simulink model "c2837xD_lcd_display"  (R2021b)
settings: Solver=FixedStepDiscrete  StartTime=0.0  StopTime=Inf  RelTol=1e-3  EnableMultiTasking=on
InitFcn:
  | c2837xD_Display_Param;
values from neighbouring files (symbols this model uses):
  SCI_counter = SCI_ping_buffer_size/SCI_chunk_size    (= 640)    [c2837xD_Display_Param.m]
  SCI_ping_buffer_size = image_height*lines_in_packet    (= 3840)    [c2837xD_Display_Param.m]
  TI_chunk_size = SCI_chunk_size    (= 6)    [c2837xD_Display_Param.m]
  TI_ping_buffer_size = SCI_ping_buffer_size    (= 3840)    [c2837xD_Display_Param.m]
libraries: c280xlib x63, c2837xDlib x63, simulink x41, c2000lib x1, demo_controls x1, dspswit3 x1, idelinklib_common x1
(part 3 of 4)

== system c2837xD_lcd_display/Initialization/GRAMWindow/Subsystem2/SetData ==
  function : TriggerPort  TriggerType=function-call  VariantControl=Variant
  Constant1 : Constant  SampleTime=-1
  Digital Output1 : c2837xDlib/Digital Output  GPIO_Number=GPIO16~GPIO23  GPIO_Bit0=off  GPIO_BIT0_Toggle=off  GPIO_Bit1=off  GPIO_BIT1_Toggle=off  GPIO_Bit2=off  GPIO_BIT2_Toggle=off  GPIO_Bit3=off  GPIO_BIT3_Toggle=off  GPIO_Bit4=off  GPIO_BIT4_Toggle=off  GPIO_Bit5=off  GPIO_BIT5_Toggle=off  GPIO_Bit6=on  GPIO_BIT6_Toggle=off  GPIO_Bit7=off  GPIO_BIT7_Toggle=off
      settings: SourceProductBaseCode=TIC2000
  wires:
  Constant1/1 -> Digital Output1/1

== system c2837xD_lcd_display/Initialization/GRAMWindow/Subsystem3/SendCommand ==
  cmd : Inport
  function : TriggerPort  TriggerType=function-call  VariantControl=Variant
  SPI Master Transfer : c280xlib/SPI Master Transfer  SPISelect=SPI_A  ClockPolarity=Rising_edge  ClockPhase=Delay_half_cycle  SPIModule=uint32(0)  Mode=Master  BusSpeed=uint32(1000000)  FirstBitToTransfer=Most significant bit (MSB)  ClockMode=0  BlockFunction=Transfer  EnableRegisterAddress=off  RegisterAddress=0  OutputDataType=int8  OutputDataLength=1  DataBits=8  UseCustomSSPin=Explicit GPIO calls  ActiveLowSSPin=Active low  Pin=124
      settings: SourceProductBaseCode=TIC2000
  Terminator : Terminator
  wires:
  cmd/1 -> SPI Master Transfer/1
  SPI Master Transfer/1 -> Terminator/1

== system c2837xD_lcd_display/Initialization/GRAMWindow/Subsystem3/SendData ==
  Data : Inport
  function : TriggerPort  TriggerType=function-call  VariantControl=Variant
  SPI Master Transfer : c280xlib/SPI Master Transfer  SPISelect=SPI_A  ClockPolarity=Rising_edge  ClockPhase=Delay_half_cycle  SPIModule=uint32(0)  Mode=Master  BusSpeed=uint32(1000000)  FirstBitToTransfer=Most significant bit (MSB)  ClockMode=0  BlockFunction=Transfer  EnableRegisterAddress=off  RegisterAddress=0  OutputDataType=int8  OutputDataLength=1  DataBits=8  UseCustomSSPin=Explicit GPIO calls  ActiveLowSSPin=Active low  Pin=124
      settings: SourceProductBaseCode=TIC2000
  Terminator : Terminator
  wires:
  Data/1 -> SPI Master Transfer/1
  SPI Master Transfer/1 -> Terminator/1

== system c2837xD_lcd_display/Initialization/GRAMWindow/Subsystem3/SetCmd ==
  function : TriggerPort  TriggerType=function-call  VariantControl=Variant
  Constant : Constant  Value=0  SampleTime=-1
  Digital Output : c2837xDlib/Digital Output  GPIO_Number=GPIO16~GPIO23  GPIO_Bit0=off  GPIO_BIT0_Toggle=off  GPIO_Bit1=off  GPIO_BIT1_Toggle=off  GPIO_Bit2=off  GPIO_BIT2_Toggle=off  GPIO_Bit3=off  GPIO_BIT3_Toggle=off  GPIO_Bit4=off  GPIO_BIT4_Toggle=off  GPIO_Bit5=off  GPIO_BIT5_Toggle=off  GPIO_Bit6=on  GPIO_BIT6_Toggle=off  GPIO_Bit7=off  GPIO_BIT7_Toggle=off
      settings: SourceProductBaseCode=TIC2000
  wires:
  Constant/1 -> Digital Output/1

== system c2837xD_lcd_display/Initialization/GRAMWindow/Subsystem3/SetData ==
  function : TriggerPort  TriggerType=function-call  VariantControl=Variant
  Constant1 : Constant  SampleTime=-1
  Digital Output1 : c2837xDlib/Digital Output  GPIO_Number=GPIO16~GPIO23  GPIO_Bit0=off  GPIO_BIT0_Toggle=off  GPIO_Bit1=off  GPIO_BIT1_Toggle=off  GPIO_Bit2=off  GPIO_BIT2_Toggle=off  GPIO_Bit3=off  GPIO_BIT3_Toggle=off  GPIO_Bit4=off  GPIO_BIT4_Toggle=off  GPIO_Bit5=off  GPIO_BIT5_Toggle=off  GPIO_Bit6=on  GPIO_BIT6_Toggle=off  GPIO_Bit7=off  GPIO_BIT7_Toggle=off
      settings: SourceProductBaseCode=TIC2000
  wires:
  Constant1/1 -> Digital Output1/1

== system c2837xD_lcd_display/Initialization/GRAMWindow/Subsystem4/SendCommand ==
  cmd : Inport
  function : TriggerPort  TriggerType=function-call  VariantControl=Variant
  SPI Master Transfer : c280xlib/SPI Master Transfer  SPISelect=SPI_A  ClockPolarity=Rising_edge  ClockPhase=Delay_half_cycle  SPIModule=uint32(0)  Mode=Master  BusSpeed=uint32(1000000)  FirstBitToTransfer=Most significant bit (MSB)  ClockMode=0  BlockFunction=Transfer  EnableRegisterAddress=off  RegisterAddress=0  OutputDataType=int8  OutputDataLength=1  DataBits=8  UseCustomSSPin=Explicit GPIO calls  ActiveLowSSPin=Active low  Pin=124
      settings: SourceProductBaseCode=TIC2000
  Terminator : Terminator
  wires:
  cmd/1 -> SPI Master Transfer/1
  SPI Master Transfer/1 -> Terminator/1

== system c2837xD_lcd_display/Initialization/GRAMWindow/Subsystem4/SendData ==
  Data : Inport
  function : TriggerPort  TriggerType=function-call  VariantControl=Variant
  SPI Master Transfer : c280xlib/SPI Master Transfer  SPISelect=SPI_A  ClockPolarity=Rising_edge  ClockPhase=Delay_half_cycle  SPIModule=uint32(0)  Mode=Master  BusSpeed=uint32(1000000)  FirstBitToTransfer=Most significant bit (MSB)  ClockMode=0  BlockFunction=Transfer  EnableRegisterAddress=off  RegisterAddress=0  OutputDataType=int8  OutputDataLength=1  DataBits=8  UseCustomSSPin=Explicit GPIO calls  ActiveLowSSPin=Active low  Pin=124
      settings: SourceProductBaseCode=TIC2000
  Terminator : Terminator
  wires:
  Data/1 -> SPI Master Transfer/1
  SPI Master Transfer/1 -> Terminator/1

== system c2837xD_lcd_display/Initialization/GRAMWindow/Subsystem4/SetCmd ==
  function : TriggerPort  TriggerType=function-call  VariantControl=Variant
  Constant : Constant  Value=0  SampleTime=-1
  Digital Output : c2837xDlib/Digital Output  GPIO_Number=GPIO16~GPIO23  GPIO_Bit0=off  GPIO_BIT0_Toggle=off  GPIO_Bit1=off  GPIO_BIT1_Toggle=off  GPIO_Bit2=off  GPIO_BIT2_Toggle=off  GPIO_Bit3=off  GPIO_BIT3_Toggle=off  GPIO_Bit4=off  GPIO_BIT4_Toggle=off  GPIO_Bit5=off  GPIO_BIT5_Toggle=off  GPIO_Bit6=on  GPIO_BIT6_Toggle=off  GPIO_Bit7=off  GPIO_BIT7_Toggle=off
      settings: SourceProductBaseCode=TIC2000
  wires:
  Constant/1 -> Digital Output/1

== system c2837xD_lcd_display/Initialization/GRAMWindow/Subsystem4/SetData ==
  function : TriggerPort  TriggerType=function-call  VariantControl=Variant
  Constant1 : Constant  SampleTime=-1
  Digital Output1 : c2837xDlib/Digital Output  GPIO_Number=GPIO16~GPIO23  GPIO_Bit0=off  GPIO_BIT0_Toggle=off  GPIO_Bit1=off  GPIO_BIT1_Toggle=off  GPIO_Bit2=off  GPIO_BIT2_Toggle=off  GPIO_Bit3=off  GPIO_BIT3_Toggle=off  GPIO_Bit4=off  GPIO_BIT4_Toggle=off  GPIO_Bit5=off  GPIO_BIT5_Toggle=off  GPIO_Bit6=on  GPIO_BIT6_Toggle=off  GPIO_Bit7=off  GPIO_BIT7_Toggle=off
      settings: SourceProductBaseCode=TIC2000
  wires:
  Constant1/1 -> Digital Output1/1

== system c2837xD_lcd_display/Initialization/GammaCorrection/Subsystem/SendCommand ==
  cmd : Inport
  function : TriggerPort  TriggerType=function-call  VariantControl=Variant
  SPI Master Transfer : c280xlib/SPI Master Transfer  SPISelect=SPI_A  ClockPolarity=Rising_edge  ClockPhase=Delay_half_cycle  SPIModule=uint32(0)  Mode=Master  BusSpeed=uint32(1000000)  FirstBitToTransfer=Most significant bit (MSB)  ClockMode=0  BlockFunction=Transfer  EnableRegisterAddress=off  RegisterAddress=0  OutputDataType=int8  OutputDataLength=1  DataBits=8  UseCustomSSPin=Explicit GPIO calls  ActiveLowSSPin=Active low  Pin=124
      settings: SourceProductBaseCode=TIC2000
  Terminator : Terminator
  wires:
  cmd/1 -> SPI Master Transfer/1
  SPI Master Transfer/1 -> Terminator/1

== system c2837xD_lcd_display/Initialization/GammaCorrection/Subsystem/SendData ==
  Data : Inport
  function : TriggerPort  TriggerType=function-call  VariantControl=Variant
  SPI Master Transfer : c280xlib/SPI Master Transfer  SPISelect=SPI_A  ClockPolarity=Rising_edge  ClockPhase=Delay_half_cycle  SPIModule=uint32(0)  Mode=Master  BusSpeed=uint32(1000000)  FirstBitToTransfer=Most significant bit (MSB)  ClockMode=0  BlockFunction=Transfer  EnableRegisterAddress=off  RegisterAddress=0  OutputDataType=int8  OutputDataLength=1  DataBits=8  UseCustomSSPin=Explicit GPIO calls  ActiveLowSSPin=Active low  Pin=124
      settings: SourceProductBaseCode=TIC2000
  Terminator : Terminator
  wires:
  Data/1 -> SPI Master Transfer/1
  SPI Master Transfer/1 -> Terminator/1

== system c2837xD_lcd_display/Initialization/GammaCorrection/Subsystem/SetCmd ==
  function : TriggerPort  TriggerType=function-call  VariantControl=Variant
  Constant : Constant  Value=0  SampleTime=-1
  Digital Output : c2837xDlib/Digital Output  GPIO_Number=GPIO16~GPIO23  GPIO_Bit0=off  GPIO_BIT0_Toggle=off  GPIO_Bit1=off  GPIO_BIT1_Toggle=off  GPIO_Bit2=off  GPIO_BIT2_Toggle=off  GPIO_Bit3=off  GPIO_BIT3_Toggle=off  GPIO_Bit4=off  GPIO_BIT4_Toggle=off  GPIO_Bit5=off  GPIO_BIT5_Toggle=off  GPIO_Bit6=on  GPIO_BIT6_Toggle=off  GPIO_Bit7=off  GPIO_BIT7_Toggle=off
      settings: SourceProductBaseCode=TIC2000
  wires:
  Constant/1 -> Digital Output/1

== system c2837xD_lcd_display/Initialization/GammaCorrection/Subsystem/SetData ==
  function : TriggerPort  TriggerType=function-call  VariantControl=Variant
  Constant1 : Constant  SampleTime=-1
  Digital Output1 : c2837xDlib/Digital Output  GPIO_Number=GPIO16~GPIO23  GPIO_Bit0=off  GPIO_BIT0_Toggle=off  GPIO_Bit1=off  GPIO_BIT1_Toggle=off  GPIO_Bit2=off  GPIO_BIT2_Toggle=off  GPIO_Bit3=off  GPIO_BIT3_Toggle=off  GPIO_Bit4=off  GPIO_BIT4_Toggle=off  GPIO_Bit5=off  GPIO_BIT5_Toggle=off  GPIO_Bit6=on  GPIO_BIT6_Toggle=off  GPIO_Bit7=off  GPIO_BIT7_Toggle=off
      settings: SourceProductBaseCode=TIC2000
  wires:
  Constant1/1 -> Digital Output1/1

== system c2837xD_lcd_display/Initialization/GammaCorrection/Subsystem1/SendCommand ==
  cmd : Inport
  function : TriggerPort  TriggerType=function-call  VariantControl=Variant
  SPI Master Transfer : c280xlib/SPI Master Transfer  SPISelect=SPI_A  ClockPolarity=Rising_edge  ClockPhase=Delay_half_cycle  SPIModule=uint32(0)  Mode=Master  BusSpeed=uint32(1000000)  FirstBitToTransfer=Most significant bit (MSB)  ClockMode=0  BlockFunction=Transfer  EnableRegisterAddress=off  RegisterAddress=0  OutputDataType=int8  OutputDataLength=1  DataBits=8  UseCustomSSPin=Explicit GPIO calls  ActiveLowSSPin=Active low  Pin=124
      settings: SourceProductBaseCode=TIC2000
  Terminator : Terminator
  wires:
  cmd/1 -> SPI Master Transfer/1
  SPI Master Transfer/1 -> Terminator/1

== system c2837xD_lcd_display/Initialization/GammaCorrection/Subsystem1/SendData ==
  Data : Inport
  function : TriggerPort  TriggerType=function-call  VariantControl=Variant
  SPI Master Transfer : c280xlib/SPI Master Transfer  SPISelect=SPI_A  ClockPolarity=Rising_edge  ClockPhase=Delay_half_cycle  SPIModule=uint32(0)  Mode=Master  BusSpeed=uint32(1000000)  FirstBitToTransfer=Most significant bit (MSB)  ClockMode=0  BlockFunction=Transfer  EnableRegisterAddress=off  RegisterAddress=0  OutputDataType=int8  OutputDataLength=1  DataBits=8  UseCustomSSPin=Explicit GPIO calls  ActiveLowSSPin=Active low  Pin=124
      settings: SourceProductBaseCode=TIC2000
  Terminator : Terminator
  wires:
  Data/1 -> SPI Master Transfer/1
  SPI Master Transfer/1 -> Terminator/1

== system c2837xD_lcd_display/Initialization/GammaCorrection/Subsystem1/SetCmd ==
  function : TriggerPort  TriggerType=function-call  VariantControl=Variant
  Constant : Constant  Value=0  SampleTime=-1
  Digital Output : c2837xDlib/Digital Output  GPIO_Number=GPIO16~GPIO23  GPIO_Bit0=off  GPIO_BIT0_Toggle=off  GPIO_Bit1=off  GPIO_BIT1_Toggle=off  GPIO_Bit2=off  GPIO_BIT2_Toggle=off  GPIO_Bit3=off  GPIO_BIT3_Toggle=off  GPIO_Bit4=off  GPIO_BIT4_Toggle=off  GPIO_Bit5=off  GPIO_BIT5_Toggle=off  GPIO_Bit6=on  GPIO_BIT6_Toggle=off  GPIO_Bit7=off  GPIO_BIT7_Toggle=off
      settings: SourceProductBaseCode=TIC2000
  wires:
  Constant/1 -> Digital Output/1

== system c2837xD_lcd_display/Initialization/GammaCorrection/Subsystem1/SetData ==
  function : TriggerPort  TriggerType=function-call  VariantControl=Variant
  Constant1 : Constant  SampleTime=-1
  Digital Output1 : c2837xDlib/Digital Output  GPIO_Number=GPIO16~GPIO23  GPIO_Bit0=off  GPIO_BIT0_Toggle=off  GPIO_Bit1=off  GPIO_BIT1_Toggle=off  GPIO_Bit2=off  GPIO_BIT2_Toggle=off  GPIO_Bit3=off  GPIO_BIT3_Toggle=off  GPIO_Bit4=off  GPIO_BIT4_Toggle=off  GPIO_Bit5=off  GPIO_BIT5_Toggle=off  GPIO_Bit6=on  GPIO_BIT6_Toggle=off  GPIO_Bit7=off  GPIO_BIT7_Toggle=off
      settings: SourceProductBaseCode=TIC2000
  wires:
  Constant1/1 -> Digital Output1/1

== system c2837xD_lcd_display/Initialization/GammaCorrection/Subsystem2/SendCommand ==
  cmd : Inport
  function : TriggerPort  TriggerType=function-call  VariantControl=Variant
  SPI Master Transfer : c280xlib/SPI Master Transfer  SPISelect=SPI_A  ClockPolarity=Rising_edge  ClockPhase=Delay_half_cycle  SPIModule=uint32(0)  Mode=Master  BusSpeed=uint32(1000000)  FirstBitToTransfer=Most significant bit (MSB)  ClockMode=0  BlockFunction=Transfer  EnableRegisterAddress=off  RegisterAddress=0  OutputDataType=int8  OutputDataLength=1  DataBits=8  UseCustomSSPin=Explicit GPIO calls  ActiveLowSSPin=Active low  Pin=124
      settings: SourceProductBaseCode=TIC2000
  Terminator : Terminator
  wires:
  cmd/1 -> SPI Master Transfer/1
  SPI Master Transfer/1 -> Terminator/1

== system c2837xD_lcd_display/Initialization/GammaCorrection/Subsystem2/SendData ==
  Data : Inport
  function : TriggerPort  TriggerType=function-call  VariantControl=Variant
  SPI Master Transfer : c280xlib/SPI Master Transfer  SPISelect=SPI_A  ClockPolarity=Rising_edge  ClockPhase=Delay_half_cycle  SPIModule=uint32(0)  Mode=Master  BusSpeed=uint32(1000000)  FirstBitToTransfer=Most significant bit (MSB)  ClockMode=0  BlockFunction=Transfer  EnableRegisterAddress=off  RegisterAddress=0  OutputDataType=int8  OutputDataLength=1  DataBits=8  UseCustomSSPin=Explicit GPIO calls  ActiveLowSSPin=Active low  Pin=124
      settings: SourceProductBaseCode=TIC2000
  Terminator : Terminator
  wires:
  Data/1 -> SPI Master Transfer/1
  SPI Master Transfer/1 -> Terminator/1

== system c2837xD_lcd_display/Initialization/GammaCorrection/Subsystem2/SetCmd ==
  function : TriggerPort  TriggerType=function-call  VariantControl=Variant
  Constant : Constant  Value=0  SampleTime=-1
  Digital Output : c2837xDlib/Digital Output  GPIO_Number=GPIO16~GPIO23  GPIO_Bit0=off  GPIO_BIT0_Toggle=off  GPIO_Bit1=off  GPIO_BIT1_Toggle=off  GPIO_Bit2=off  GPIO_BIT2_Toggle=off  GPIO_Bit3=off  GPIO_BIT3_Toggle=off  GPIO_Bit4=off  GPIO_BIT4_Toggle=off  GPIO_Bit5=off  GPIO_BIT5_Toggle=off  GPIO_Bit6=on  GPIO_BIT6_Toggle=off  GPIO_Bit7=off  GPIO_BIT7_Toggle=off
      settings: SourceProductBaseCode=TIC2000
  wires:
  Constant/1 -> Digital Output/1

== system c2837xD_lcd_display/Initialization/GammaCorrection/Subsystem2/SetData ==
  function : TriggerPort  TriggerType=function-call  VariantControl=Variant
  Constant1 : Constant  SampleTime=-1
  Digital Output1 : c2837xDlib/Digital Output  GPIO_Number=GPIO16~GPIO23  GPIO_Bit0=off  GPIO_BIT0_Toggle=off  GPIO_Bit1=off  GPIO_BIT1_Toggle=off  GPIO_Bit2=off  GPIO_BIT2_Toggle=off  GPIO_Bit3=off  GPIO_BIT3_Toggle=off  GPIO_Bit4=off  GPIO_BIT4_Toggle=off  GPIO_Bit5=off  GPIO_BIT5_Toggle=off  GPIO_Bit6=on  GPIO_BIT6_Toggle=off  GPIO_Bit7=off  GPIO_BIT7_Toggle=off
      settings: SourceProductBaseCode=TIC2000
  wires:
  Constant1/1 -> Digital Output1/1

== system c2837xD_lcd_display/Initialization/GammaCorrection/Subsystem3/SendCommand ==
  cmd : Inport
  function : TriggerPort  TriggerType=function-call  VariantControl=Variant
  SPI Master Transfer : c280xlib/SPI Master Transfer  SPISelect=SPI_A  ClockPolarity=Rising_edge  ClockPhase=Delay_half_cycle  SPIModule=uint32(0)  Mode=Master  BusSpeed=uint32(1000000)  FirstBitToTransfer=Most significant bit (MSB)  ClockMode=0  BlockFunction=Transfer  EnableRegisterAddress=off  RegisterAddress=0  OutputDataType=int8  OutputDataLength=1  DataBits=8  UseCustomSSPin=Explicit GPIO calls  ActiveLowSSPin=Active low  Pin=124
      settings: SourceProductBaseCode=TIC2000
  Terminator : Terminator
  wires:
  cmd/1 -> SPI Master Transfer/1
  SPI Master Transfer/1 -> Terminator/1

== system c2837xD_lcd_display/Initialization/GammaCorrection/Subsystem3/SendData ==
  Data : Inport
  function : TriggerPort  TriggerType=function-call  VariantControl=Variant
  SPI Master Transfer : c280xlib/SPI Master Transfer  SPISelect=SPI_A  ClockPolarity=Rising_edge  ClockPhase=Delay_half_cycle  SPIModule=uint32(0)  Mode=Master  BusSpeed=uint32(1000000)  FirstBitToTransfer=Most significant bit (MSB)  ClockMode=0  BlockFunction=Transfer  EnableRegisterAddress=off  RegisterAddress=0  OutputDataType=int8  OutputDataLength=1  DataBits=8  UseCustomSSPin=Explicit GPIO calls  ActiveLowSSPin=Active low  Pin=124
      settings: SourceProductBaseCode=TIC2000
  Terminator : Terminator
  wires:
  Data/1 -> SPI Master Transfer/1
  SPI Master Transfer/1 -> Terminator/1

== system c2837xD_lcd_display/Initialization/GammaCorrection/Subsystem3/SetCmd ==
  function : TriggerPort  TriggerType=function-call  VariantControl=Variant
  Constant : Constant  Value=0  SampleTime=-1
  Digital Output : c2837xDlib/Digital Output  GPIO_Number=GPIO16~GPIO23  GPIO_Bit0=off  GPIO_BIT0_Toggle=off  GPIO_Bit1=off  GPIO_BIT1_Toggle=off  GPIO_Bit2=off  GPIO_BIT2_Toggle=off  GPIO_Bit3=off  GPIO_BIT3_Toggle=off  GPIO_Bit4=off  GPIO_BIT4_Toggle=off  GPIO_Bit5=off  GPIO_BIT5_Toggle=off  GPIO_Bit6=on  GPIO_BIT6_Toggle=off  GPIO_Bit7=off  GPIO_BIT7_Toggle=off
      settings: SourceProductBaseCode=TIC2000
  wires:
  Constant/1 -> Digital Output/1

== system c2837xD_lcd_display/Initialization/GammaCorrection/Subsystem3/SetData ==
  function : TriggerPort  TriggerType=function-call  VariantControl=Variant
  Constant1 : Constant  SampleTime=-1
  Digital Output1 : c2837xDlib/Digital Output  GPIO_Number=GPIO16~GPIO23  GPIO_Bit0=off  GPIO_BIT0_Toggle=off  GPIO_Bit1=off  GPIO_BIT1_Toggle=off  GPIO_Bit2=off  GPIO_BIT2_Toggle=off  GPIO_Bit3=off  GPIO_BIT3_Toggle=off  GPIO_Bit4=off  GPIO_BIT4_Toggle=off  GPIO_Bit5=off  GPIO_BIT5_Toggle=off  GPIO_Bit6=on  GPIO_BIT6_Toggle=off  GPIO_Bit7=off  GPIO_BIT7_Toggle=off
      settings: SourceProductBaseCode=TIC2000
  wires:
  Constant1/1 -> Digital Output1/1

== system c2837xD_lcd_display/Initialization/GammaCorrection/Subsystem4/SendCommand ==
  cmd : Inport
  function : TriggerPort  TriggerType=function-call  VariantControl=Variant
  SPI Master Transfer : c280xlib/SPI Master Transfer  SPISelect=SPI_A  ClockPolarity=Rising_edge  ClockPhase=Delay_half_cycle  SPIModule=uint32(0)  Mode=Master  BusSpeed=uint32(1000000)  FirstBitToTransfer=Most significant bit (MSB)  ClockMode=0  BlockFunction=Transfer  EnableRegisterAddress=off  RegisterAddress=0  OutputDataType=int8  OutputDataLength=1  DataBits=8  UseCustomSSPin=Explicit GPIO calls  ActiveLowSSPin=Active low  Pin=124
      settings: SourceProductBaseCode=TIC2000
  Terminator : Terminator
  wires:
  cmd/1 -> SPI Master Transfer/1
  SPI Master Transfer/1 -> Terminator/1

== system c2837xD_lcd_display/Initialization/GammaCorrection/Subsystem4/SendData ==
  Data : Inport
  function : TriggerPort  TriggerType=function-call  VariantControl=Variant
  SPI Master Transfer : c280xlib/SPI Master Transfer  SPISelect=SPI_A  ClockPolarity=Rising_edge  ClockPhase=Delay_half_cycle  SPIModule=uint32(0)  Mode=Master  BusSpeed=uint32(1000000)  FirstBitToTransfer=Most significant bit (MSB)  ClockMode=0  BlockFunction=Transfer  EnableRegisterAddress=off  RegisterAddress=0  OutputDataType=int8  OutputDataLength=1  DataBits=8  UseCustomSSPin=Explicit GPIO calls  ActiveLowSSPin=Active low  Pin=124
      settings: SourceProductBaseCode=TIC2000
  Terminator : Terminator
  wires:
  Data/1 -> SPI Master Transfer/1
  SPI Master Transfer/1 -> Terminator/1

== system c2837xD_lcd_display/Initialization/GammaCorrection/Subsystem4/SetCmd ==
  function : TriggerPort  TriggerType=function-call  VariantControl=Variant
  Constant : Constant  Value=0  SampleTime=-1
  Digital Output : c2837xDlib/Digital Output  GPIO_Number=GPIO16~GPIO23  GPIO_Bit0=off  GPIO_BIT0_Toggle=off  GPIO_Bit1=off  GPIO_BIT1_Toggle=off  GPIO_Bit2=off  GPIO_BIT2_Toggle=off  GPIO_Bit3=off  GPIO_BIT3_Toggle=off  GPIO_Bit4=off  GPIO_BIT4_Toggle=off  GPIO_Bit5=off  GPIO_BIT5_Toggle=off  GPIO_Bit6=on  GPIO_BIT6_Toggle=off  GPIO_Bit7=off  GPIO_BIT7_Toggle=off
      settings: SourceProductBaseCode=TIC2000
  wires:
  Constant/1 -> Digital Output/1

== system c2837xD_lcd_display/Initialization/GammaCorrection/Subsystem4/SetData ==
  function : TriggerPort  TriggerType=function-call  VariantControl=Variant
  Constant1 : Constant  SampleTime=-1
  Digital Output1 : c2837xDlib/Digital Output  GPIO_Number=GPIO16~GPIO23  GPIO_Bit0=off  GPIO_BIT0_Toggle=off  GPIO_Bit1=off  GPIO_BIT1_Toggle=off  GPIO_Bit2=off  GPIO_BIT2_Toggle=off  GPIO_Bit3=off  GPIO_BIT3_Toggle=off  GPIO_Bit4=off  GPIO_BIT4_Toggle=off  GPIO_Bit5=off  GPIO_BIT5_Toggle=off  GPIO_Bit6=on  GPIO_BIT6_Toggle=off  GPIO_Bit7=off  GPIO_BIT7_Toggle=off
      settings: SourceProductBaseCode=TIC2000
  wires:
  Constant1/1 -> Digital Output1/1

== system c2837xD_lcd_display/Initialization/GammaCorrection1/Subsystem/SendCommand ==
  cmd : Inport
  function : TriggerPort  TriggerType=function-call  VariantControl=Variant
  SPI Master Transfer : c280xlib/SPI Master Transfer  SPISelect=SPI_A  ClockPolarity=Rising_edge  ClockPhase=Delay_half_cycle  SPIModule=uint32(0)  Mode=Master  BusSpeed=uint32(1000000)  FirstBitToTransfer=Most significant bit (MSB)  ClockMode=0  BlockFunction=Transfer  EnableRegisterAddress=off  RegisterAddress=0  OutputDataType=int8  OutputDataLength=1  DataBits=8  UseCustomSSPin=Explicit GPIO calls  ActiveLowSSPin=Active low  Pin=124
      settings: SourceProductBaseCode=TIC2000
  Terminator : Terminator
  wires:
  cmd/1 -> SPI Master Transfer/1
  SPI Master Transfer/1 -> Terminator/1

== system c2837xD_lcd_display/Initialization/GammaCorrection1/Subsystem/SendData ==
  Data : Inport
  function : TriggerPort  TriggerType=function-call  VariantControl=Variant
  SPI Master Transfer : c280xlib/SPI Master Transfer  SPISelect=SPI_A  ClockPolarity=Rising_edge  ClockPhase=Delay_half_cycle  SPIModule=uint32(0)  Mode=Master  BusSpeed=uint32(1000000)  FirstBitToTransfer=Most significant bit (MSB)  ClockMode=0  BlockFunction=Transfer  EnableRegisterAddress=off  RegisterAddress=0  OutputDataType=int8  OutputDataLength=1  DataBits=8  UseCustomSSPin=Explicit GPIO calls  ActiveLowSSPin=Active low  Pin=124
      settings: SourceProductBaseCode=TIC2000
  Terminator : Terminator
  wires:
  Data/1 -> SPI Master Transfer/1
  SPI Master Transfer/1 -> Terminator/1

== system c2837xD_lcd_display/Initialization/GammaCorrection1/Subsystem/SetCmd ==
  function : TriggerPort  TriggerType=function-call  VariantControl=Variant
  Constant : Constant  Value=0  SampleTime=-1
  Digital Output : c2837xDlib/Digital Output  GPIO_Number=GPIO16~GPIO23  GPIO_Bit0=off  GPIO_BIT0_Toggle=off  GPIO_Bit1=off  GPIO_BIT1_Toggle=off  GPIO_Bit2=off  GPIO_BIT2_Toggle=off  GPIO_Bit3=off  GPIO_BIT3_Toggle=off  GPIO_Bit4=off  GPIO_BIT4_Toggle=off  GPIO_Bit5=off  GPIO_BIT5_Toggle=off  GPIO_Bit6=on  GPIO_BIT6_Toggle=off  GPIO_Bit7=off  GPIO_BIT7_Toggle=off
      settings: SourceProductBaseCode=TIC2000
  wires:
  Constant/1 -> Digital Output/1

== system c2837xD_lcd_display/Initialization/GammaCorrection1/Subsystem/SetData ==
  function : TriggerPort  TriggerType=function-call  VariantControl=Variant
  Constant1 : Constant  SampleTime=-1
  Digital Output1 : c2837xDlib/Digital Output  GPIO_Number=GPIO16~GPIO23  GPIO_Bit0=off  GPIO_BIT0_Toggle=off  GPIO_Bit1=off  GPIO_BIT1_Toggle=off  GPIO_Bit2=off  GPIO_BIT2_Toggle=off  GPIO_Bit3=off  GPIO_BIT3_Toggle=off  GPIO_Bit4=off  GPIO_BIT4_Toggle=off  GPIO_Bit5=off  GPIO_BIT5_Toggle=off  GPIO_Bit6=on  GPIO_BIT6_Toggle=off  GPIO_Bit7=off  GPIO_BIT7_Toggle=off
      settings: SourceProductBaseCode=TIC2000
  wires:
  Constant1/1 -> Digital Output1/1

== system c2837xD_lcd_display/Initialization/GammaCorrection1/Subsystem1/SendCommand ==
  cmd : Inport
  function : TriggerPort  TriggerType=function-call  VariantControl=Variant
  SPI Master Transfer : c280xlib/SPI Master Transfer  SPISelect=SPI_A  ClockPolarity=Rising_edge  ClockPhase=Delay_half_cycle  SPIModule=uint32(0)  Mode=Master  BusSpeed=uint32(1000000)  FirstBitToTransfer=Most significant bit (MSB)  ClockMode=0  BlockFunction=Transfer  EnableRegisterAddress=off  RegisterAddress=0  OutputDataType=int8  OutputDataLength=1  DataBits=8  UseCustomSSPin=Explicit GPIO calls  ActiveLowSSPin=Active low  Pin=124
      settings: SourceProductBaseCode=TIC2000
  Terminator : Terminator
  wires:
  cmd/1 -> SPI Master Transfer/1
  SPI Master Transfer/1 -> Terminator/1

== system c2837xD_lcd_display/Initialization/GammaCorrection1/Subsystem1/SendData ==
  Data : Inport
  function : TriggerPort  TriggerType=function-call  VariantControl=Variant
  SPI Master Transfer : c280xlib/SPI Master Transfer  SPISelect=SPI_A  ClockPolarity=Rising_edge  ClockPhase=Delay_half_cycle  SPIModule=uint32(0)  Mode=Master  BusSpeed=uint32(1000000)  FirstBitToTransfer=Most significant bit (MSB)  ClockMode=0  BlockFunction=Transfer  EnableRegisterAddress=off  RegisterAddress=0  OutputDataType=int8  OutputDataLength=1  DataBits=8  UseCustomSSPin=Explicit GPIO calls  ActiveLowSSPin=Active low  Pin=124
      settings: SourceProductBaseCode=TIC2000
  Terminator : Terminator
  wires:
  Data/1 -> SPI Master Transfer/1
  SPI Master Transfer/1 -> Terminator/1

== system c2837xD_lcd_display/Initialization/GammaCorrection1/Subsystem1/SetCmd ==
  function : TriggerPort  TriggerType=function-call  VariantControl=Variant
  Constant : Constant  Value=0  SampleTime=-1
  Digital Output : c2837xDlib/Digital Output  GPIO_Number=GPIO16~GPIO23  GPIO_Bit0=off  GPIO_BIT0_Toggle=off  GPIO_Bit1=off  GPIO_BIT1_Toggle=off  GPIO_Bit2=off  GPIO_BIT2_Toggle=off  GPIO_Bit3=off  GPIO_BIT3_Toggle=off  GPIO_Bit4=off  GPIO_BIT4_Toggle=off  GPIO_Bit5=off  GPIO_BIT5_Toggle=off  GPIO_Bit6=on  GPIO_BIT6_Toggle=off  GPIO_Bit7=off  GPIO_BIT7_Toggle=off
      settings: SourceProductBaseCode=TIC2000
  wires:
  Constant/1 -> Digital Output/1

== system c2837xD_lcd_display/Initialization/GammaCorrection1/Subsystem1/SetData ==
  function : TriggerPort  TriggerType=function-call  VariantControl=Variant
  Constant1 : Constant  SampleTime=-1
  Digital Output1 : c2837xDlib/Digital Output  GPIO_Number=GPIO16~GPIO23  GPIO_Bit0=off  GPIO_BIT0_Toggle=off  GPIO_Bit1=off  GPIO_BIT1_Toggle=off  GPIO_Bit2=off  GPIO_BIT2_Toggle=off  GPIO_Bit3=off  GPIO_BIT3_Toggle=off  GPIO_Bit4=off  GPIO_BIT4_Toggle=off  GPIO_Bit5=off  GPIO_BIT5_Toggle=off  GPIO_Bit6=on  GPIO_BIT6_Toggle=off  GPIO_Bit7=off  GPIO_BIT7_Toggle=off
      settings: SourceProductBaseCode=TIC2000
  wires:
  Constant1/1 -> Digital Output1/1

== system c2837xD_lcd_display/Initialization/GammaCorrection1/Subsystem2/SendCommand ==
  cmd : Inport
  function : TriggerPort  TriggerType=function-call  VariantControl=Variant
  SPI Master Transfer : c280xlib/SPI Master Transfer  SPISelect=SPI_A  ClockPolarity=Rising_edge  ClockPhase=Delay_half_cycle  SPIModule=uint32(0)  Mode=Master  BusSpeed=uint32(1000000)  FirstBitToTransfer=Most significant bit (MSB)  ClockMode=0  BlockFunction=Transfer  EnableRegisterAddress=off  RegisterAddress=0  OutputDataType=int8  OutputDataLength=1  DataBits=8  UseCustomSSPin=Explicit GPIO calls  ActiveLowSSPin=Active low  Pin=124
      settings: SourceProductBaseCode=TIC2000
  Terminator : Terminator
  wires:
  cmd/1 -> SPI Master Transfer/1
  SPI Master Transfer/1 -> Terminator/1

== system c2837xD_lcd_display/Initialization/GammaCorrection1/Subsystem2/SendData ==
  Data : Inport
  function : TriggerPort  TriggerType=function-call  VariantControl=Variant
  SPI Master Transfer : c280xlib/SPI Master Transfer  SPISelect=SPI_A  ClockPolarity=Rising_edge  ClockPhase=Delay_half_cycle  SPIModule=uint32(0)  Mode=Master  BusSpeed=uint32(1000000)  FirstBitToTransfer=Most significant bit (MSB)  ClockMode=0  BlockFunction=Transfer  EnableRegisterAddress=off  RegisterAddress=0  OutputDataType=int8  OutputDataLength=1  DataBits=8  UseCustomSSPin=Explicit GPIO calls  ActiveLowSSPin=Active low  Pin=124
      settings: SourceProductBaseCode=TIC2000
  Terminator : Terminator
  wires:
  Data/1 -> SPI Master Transfer/1
  SPI Master Transfer/1 -> Terminator/1

== system c2837xD_lcd_display/Initialization/GammaCorrection1/Subsystem2/SetCmd ==
  function : TriggerPort  TriggerType=function-call  VariantControl=Variant
  Constant : Constant  Value=0  SampleTime=-1
  Digital Output : c2837xDlib/Digital Output  GPIO_Number=GPIO16~GPIO23  GPIO_Bit0=off  GPIO_BIT0_Toggle=off  GPIO_Bit1=off  GPIO_BIT1_Toggle=off  GPIO_Bit2=off  GPIO_BIT2_Toggle=off  GPIO_Bit3=off  GPIO_BIT3_Toggle=off  GPIO_Bit4=off  GPIO_BIT4_Toggle=off  GPIO_Bit5=off  GPIO_BIT5_Toggle=off  GPIO_Bit6=on  GPIO_BIT6_Toggle=off  GPIO_Bit7=off  GPIO_BIT7_Toggle=off
      settings: SourceProductBaseCode=TIC2000
  wires:
  Constant/1 -> Digital Output/1

== system c2837xD_lcd_display/Initialization/GammaCorrection1/Subsystem2/SetData ==
  function : TriggerPort  TriggerType=function-call  VariantControl=Variant
  Constant1 : Constant  SampleTime=-1
  Digital Output1 : c2837xDlib/Digital Output  GPIO_Number=GPIO16~GPIO23  GPIO_Bit0=off  GPIO_BIT0_Toggle=off  GPIO_Bit1=off  GPIO_BIT1_Toggle=off  GPIO_Bit2=off  GPIO_BIT2_Toggle=off  GPIO_Bit3=off  GPIO_BIT3_Toggle=off  GPIO_Bit4=off  GPIO_BIT4_Toggle=off  GPIO_Bit5=off  GPIO_BIT5_Toggle=off  GPIO_Bit6=on  GPIO_BIT6_Toggle=off  GPIO_Bit7=off  GPIO_BIT7_Toggle=off
      settings: SourceProductBaseCode=TIC2000
  wires:
  Constant1/1 -> Digital Output1/1

== system c2837xD_lcd_display/Initialization/GammaCorrection1/Subsystem3/SendCommand ==
  cmd : Inport
  function : TriggerPort  TriggerType=function-call  VariantControl=Variant
  SPI Master Transfer : c280xlib/SPI Master Transfer  SPISelect=SPI_A  ClockPolarity=Rising_edge  ClockPhase=Delay_half_cycle  SPIModule=uint32(0)  Mode=Master  BusSpeed=uint32(1000000)  FirstBitToTransfer=Most significant bit (MSB)  ClockMode=0  BlockFunction=Transfer  EnableRegisterAddress=off  RegisterAddress=0  OutputDataType=int8  OutputDataLength=1  DataBits=8  UseCustomSSPin=Explicit GPIO calls  ActiveLowSSPin=Active low  Pin=124
      settings: SourceProductBaseCode=TIC2000
  Terminator : Terminator
  wires:
  cmd/1 -> SPI Master Transfer/1
  SPI Master Transfer/1 -> Terminator/1

== system c2837xD_lcd_display/Initialization/GammaCorrection1/Subsystem3/SendData ==
  Data : Inport
  function : TriggerPort  TriggerType=function-call  VariantControl=Variant
  SPI Master Transfer : c280xlib/SPI Master Transfer  SPISelect=SPI_A  ClockPolarity=Rising_edge  ClockPhase=Delay_half_cycle  SPIModule=uint32(0)  Mode=Master  BusSpeed=uint32(1000000)  FirstBitToTransfer=Most significant bit (MSB)  ClockMode=0  BlockFunction=Transfer  EnableRegisterAddress=off  RegisterAddress=0  OutputDataType=int8  OutputDataLength=1  DataBits=8  UseCustomSSPin=Explicit GPIO calls  ActiveLowSSPin=Active low  Pin=124
      settings: SourceProductBaseCode=TIC2000
  Terminator : Terminator
  wires:
  Data/1 -> SPI Master Transfer/1
  SPI Master Transfer/1 -> Terminator/1

== system c2837xD_lcd_display/Initialization/GammaCorrection1/Subsystem3/SetCmd ==
  function : TriggerPort  TriggerType=function-call  VariantControl=Variant
  Constant : Constant  Value=0  SampleTime=-1
  Digital Output : c2837xDlib/Digital Output  GPIO_Number=GPIO16~GPIO23  GPIO_Bit0=off  GPIO_BIT0_Toggle=off  GPIO_Bit1=off  GPIO_BIT1_Toggle=off  GPIO_Bit2=off  GPIO_BIT2_Toggle=off  GPIO_Bit3=off  GPIO_BIT3_Toggle=off  GPIO_Bit4=off  GPIO_BIT4_Toggle=off  GPIO_Bit5=off  GPIO_BIT5_Toggle=off  GPIO_Bit6=on  GPIO_BIT6_Toggle=off  GPIO_Bit7=off  GPIO_BIT7_Toggle=off
      settings: SourceProductBaseCode=TIC2000
  wires:
  Constant/1 -> Digital Output/1

== system c2837xD_lcd_display/Initialization/GammaCorrection1/Subsystem3/SetData ==
  function : TriggerPort  TriggerType=function-call  VariantControl=Variant
  Constant1 : Constant  SampleTime=-1
  Digital Output1 : c2837xDlib/Digital Output  GPIO_Number=GPIO16~GPIO23  GPIO_Bit0=off  GPIO_BIT0_Toggle=off  GPIO_Bit1=off  GPIO_BIT1_Toggle=off  GPIO_Bit2=off  GPIO_BIT2_Toggle=off  GPIO_Bit3=off  GPIO_BIT3_Toggle=off  GPIO_Bit4=off  GPIO_BIT4_Toggle=off  GPIO_Bit5=off  GPIO_BIT5_Toggle=off  GPIO_Bit6=on  GPIO_BIT6_Toggle=off  GPIO_Bit7=off  GPIO_BIT7_Toggle=off
      settings: SourceProductBaseCode=TIC2000
  wires:
  Constant1/1 -> Digital Output1/1

== system c2837xD_lcd_display/Initialization/GammaCorrection1/Subsystem4/SendCommand ==
  cmd : Inport
  function : TriggerPort  TriggerType=function-call  VariantControl=Variant
  SPI Master Transfer : c280xlib/SPI Master Transfer  SPISelect=SPI_A  ClockPolarity=Rising_edge  ClockPhase=Delay_half_cycle  SPIModule=uint32(0)  Mode=Master  BusSpeed=uint32(1000000)  FirstBitToTransfer=Most significant bit (MSB)  ClockMode=0  BlockFunction=Transfer  EnableRegisterAddress=off  RegisterAddress=0  OutputDataType=int8  OutputDataLength=1  DataBits=8  UseCustomSSPin=Explicit GPIO calls  ActiveLowSSPin=Active low  Pin=124
      settings: SourceProductBaseCode=TIC2000
  Terminator : Terminator
  wires:
  cmd/1 -> SPI Master Transfer/1
  SPI Master Transfer/1 -> Terminator/1

== system c2837xD_lcd_display/Initialization/GammaCorrection1/Subsystem4/SendData ==
  Data : Inport
  function : TriggerPort  TriggerType=function-call  VariantControl=Variant
  SPI Master Transfer : c280xlib/SPI Master Transfer  SPISelect=SPI_A  ClockPolarity=Rising_edge  ClockPhase=Delay_half_cycle  SPIModule=uint32(0)  Mode=Master  BusSpeed=uint32(1000000)  FirstBitToTransfer=Most significant bit (MSB)  ClockMode=0  BlockFunction=Transfer  EnableRegisterAddress=off  RegisterAddress=0  OutputDataType=int8  OutputDataLength=1  DataBits=8  UseCustomSSPin=Explicit GPIO calls  ActiveLowSSPin=Active low  Pin=124
      settings: SourceProductBaseCode=TIC2000
  Terminator : Terminator
  wires:
  Data/1 -> SPI Master Transfer/1
  SPI Master Transfer/1 -> Terminator/1

== system c2837xD_lcd_display/Initialization/GammaCorrection1/Subsystem4/SetCmd ==
  function : TriggerPort  TriggerType=function-call  VariantControl=Variant
  Constant : Constant  Value=0  SampleTime=-1
  Digital Output : c2837xDlib/Digital Output  GPIO_Number=GPIO16~GPIO23  GPIO_Bit0=off  GPIO_BIT0_Toggle=off  GPIO_Bit1=off  GPIO_BIT1_Toggle=off  GPIO_Bit2=off  GPIO_BIT2_Toggle=off  GPIO_Bit3=off  GPIO_BIT3_Toggle=off  GPIO_Bit4=off  GPIO_BIT4_Toggle=off  GPIO_Bit5=off  GPIO_BIT5_Toggle=off  GPIO_Bit6=on  GPIO_BIT6_Toggle=off  GPIO_Bit7=off  GPIO_BIT7_Toggle=off
      settings: SourceProductBaseCode=TIC2000
  wires:
  Constant/1 -> Digital Output/1

== system c2837xD_lcd_display/Initialization/GammaCorrection1/Subsystem4/SetData ==
  function : TriggerPort  TriggerType=function-call  VariantControl=Variant
  Constant1 : Constant  SampleTime=-1
  Digital Output1 : c2837xDlib/Digital Output  GPIO_Number=GPIO16~GPIO23  GPIO_Bit0=off  GPIO_BIT0_Toggle=off  GPIO_Bit1=off  GPIO_BIT1_Toggle=off  GPIO_Bit2=off  GPIO_BIT2_Toggle=off  GPIO_Bit3=off  GPIO_BIT3_Toggle=off  GPIO_Bit4=off  GPIO_BIT4_Toggle=off  GPIO_Bit5=off  GPIO_BIT5_Toggle=off  GPIO_Bit6=on  GPIO_BIT6_Toggle=off  GPIO_Bit7=off  GPIO_BIT7_Toggle=off
      settings: SourceProductBaseCode=TIC2000
  wires:
  Constant1/1 -> Digital Output1/1

== system c2837xD_lcd_display/Initialization/InitPwr/Subsystem/SendCommand ==
  cmd : Inport
  function : TriggerPort  TriggerType=function-call  VariantControl=Variant
  SPI Master Transfer : c280xlib/SPI Master Transfer  SPISelect=SPI_A  ClockPolarity=Rising_edge  ClockPhase=Delay_half_cycle  SPIModule=uint32(0)  Mode=Master  BusSpeed=uint32(1000000)  FirstBitToTransfer=Most significant bit (MSB)  ClockMode=0  BlockFunction=Transfer  EnableRegisterAddress=off  RegisterAddress=0  OutputDataType=int8  OutputDataLength=1  DataBits=8  UseCustomSSPin=Explicit GPIO calls  ActiveLowSSPin=Active low  Pin=124
      settings: SourceProductBaseCode=TIC2000
  Terminator : Terminator
  wires:
  cmd/1 -> SPI Master Transfer/1
  SPI Master Transfer/1 -> Terminator/1

== system c2837xD_lcd_display/Initialization/InitPwr/Subsystem/SendData ==
  Data : Inport
  function : TriggerPort  TriggerType=function-call  VariantControl=Variant
  SPI Master Transfer : c280xlib/SPI Master Transfer  SPISelect=SPI_A  ClockPolarity=Rising_edge  ClockPhase=Delay_half_cycle  SPIModule=uint32(0)  Mode=Master  BusSpeed=uint32(1000000)  FirstBitToTransfer=Most significant bit (MSB)  ClockMode=0  BlockFunction=Transfer  EnableRegisterAddress=off  RegisterAddress=0  OutputDataType=int8  OutputDataLength=1  DataBits=8  UseCustomSSPin=Explicit GPIO calls  ActiveLowSSPin=Active low  Pin=124
      settings: SourceProductBaseCode=TIC2000
  Terminator : Terminator
  wires:
  Data/1 -> SPI Master Transfer/1
  SPI Master Transfer/1 -> Terminator/1

== system c2837xD_lcd_display/Initialization/InitPwr/Subsystem/SetCmd ==
  function : TriggerPort  TriggerType=function-call  VariantControl=Variant
  Constant : Constant  Value=0  SampleTime=-1
  Digital Output : c2837xDlib/Digital Output  GPIO_Number=GPIO16~GPIO23  GPIO_Bit0=off  GPIO_BIT0_Toggle=off  GPIO_Bit1=off  GPIO_BIT1_Toggle=off  GPIO_Bit2=off  GPIO_BIT2_Toggle=off  GPIO_Bit3=off  GPIO_BIT3_Toggle=off  GPIO_Bit4=off  GPIO_BIT4_Toggle=off  GPIO_Bit5=off  GPIO_BIT5_Toggle=off  GPIO_Bit6=on  GPIO_BIT6_Toggle=off  GPIO_Bit7=off  GPIO_BIT7_Toggle=off
      settings: SourceProductBaseCode=TIC2000
  wires:
  Constant/1 -> Digital Output/1

== system c2837xD_lcd_display/Initialization/InitPwr/Subsystem/SetData ==
  function : TriggerPort  TriggerType=function-call  VariantControl=Variant
  Constant1 : Constant  SampleTime=-1
  Digital Output1 : c2837xDlib/Digital Output  GPIO_Number=GPIO16~GPIO23  GPIO_Bit0=off  GPIO_BIT0_Toggle=off  GPIO_Bit1=off  GPIO_BIT1_Toggle=off  GPIO_Bit2=off  GPIO_BIT2_Toggle=off  GPIO_Bit3=off  GPIO_BIT3_Toggle=off  GPIO_Bit4=off  GPIO_BIT4_Toggle=off  GPIO_Bit5=off  GPIO_BIT5_Toggle=off  GPIO_Bit6=on  GPIO_BIT6_Toggle=off  GPIO_Bit7=off  GPIO_BIT7_Toggle=off
      settings: SourceProductBaseCode=TIC2000
  wires:
  Constant1/1 -> Digital Output1/1

== system c2837xD_lcd_display/Initialization/OUTPUT_CTRL_REG/Subsystem/SendCommand ==
  cmd : Inport
  function : TriggerPort  TriggerType=function-call  VariantControl=Variant
  SPI Master Transfer : c280xlib/SPI Master Transfer  SPISelect=SPI_A  ClockPolarity=Rising_edge  ClockPhase=Delay_half_cycle  SPIModule=uint32(0)  Mode=Master  BusSpeed=uint32(1000000)  FirstBitToTransfer=Most significant bit (MSB)  ClockMode=0  BlockFunction=Transfer  EnableRegisterAddress=off  RegisterAddress=0  OutputDataType=int8  OutputDataLength=1  DataBits=8  UseCustomSSPin=Explicit GPIO calls  ActiveLowSSPin=Active low  Pin=124
      settings: SourceProductBaseCode=TIC2000
  Terminator : Terminator
  wires:
  cmd/1 -> SPI Master Transfer/1
  SPI Master Transfer/1 -> Terminator/1

== system c2837xD_lcd_display/Initialization/OUTPUT_CTRL_REG/Subsystem/SendData ==
  Data : Inport
  function : TriggerPort  TriggerType=function-call  VariantControl=Variant
  SPI Master Transfer : c280xlib/SPI Master Transfer  SPISelect=SPI_A  ClockPolarity=Rising_edge  ClockPhase=Delay_half_cycle  SPIModule=uint32(0)  Mode=Master  BusSpeed=uint32(1000000)  FirstBitToTransfer=Most significant bit (MSB)  ClockMode=0  BlockFunction=Transfer  EnableRegisterAddress=off  RegisterAddress=0  OutputDataType=int8  OutputDataLength=1  DataBits=8  UseCustomSSPin=Explicit GPIO calls  ActiveLowSSPin=Active low  Pin=124
      settings: SourceProductBaseCode=TIC2000
  Terminator : Terminator
  wires:
  Data/1 -> SPI Master Transfer/1
  SPI Master Transfer/1 -> Terminator/1

== system c2837xD_lcd_display/Initialization/OUTPUT_CTRL_REG/Subsystem/SetCmd ==
  function : TriggerPort  TriggerType=function-call  VariantControl=Variant
  Constant : Constant  Value=0  SampleTime=-1
  Digital Output : c2837xDlib/Digital Output  GPIO_Number=GPIO16~GPIO23  GPIO_Bit0=off  GPIO_BIT0_Toggle=off  GPIO_Bit1=off  GPIO_BIT1_Toggle=off  GPIO_Bit2=off  GPIO_BIT2_Toggle=off  GPIO_Bit3=off  GPIO_BIT3_Toggle=off  GPIO_Bit4=off  GPIO_BIT4_Toggle=off  GPIO_Bit5=off  GPIO_BIT5_Toggle=off  GPIO_Bit6=on  GPIO_BIT6_Toggle=off  GPIO_Bit7=off  GPIO_BIT7_Toggle=off
      settings: SourceProductBaseCode=TIC2000
  wires:
  Constant/1 -> Digital Output/1

== system c2837xD_lcd_display/Initialization/OUTPUT_CTRL_REG/Subsystem/SetData ==
  function : TriggerPort  TriggerType=function-call  VariantControl=Variant
  Constant1 : Constant  SampleTime=-1
  Digital Output1 : c2837xDlib/Digital Output  GPIO_Number=GPIO16~GPIO23  GPIO_Bit0=off  GPIO_BIT0_Toggle=off  GPIO_Bit1=off  GPIO_BIT1_Toggle=off  GPIO_Bit2=off  GPIO_BIT2_Toggle=off  GPIO_Bit3=off  GPIO_BIT3_Toggle=off  GPIO_Bit4=off  GPIO_BIT4_Toggle=off  GPIO_Bit5=off  GPIO_BIT5_Toggle=off  GPIO_Bit6=on  GPIO_BIT6_Toggle=off  GPIO_Bit7=off  GPIO_BIT7_Toggle=off
      settings: SourceProductBaseCode=TIC2000
  wires:
  Constant1/1 -> Digital Output1/1

== system c2837xD_lcd_display/Initialization/OscStart/Subsystem/SendCommand ==
  cmd : Inport
  function : TriggerPort  TriggerType=function-call  VariantControl=Variant
  SPI Master Transfer : c280xlib/SPI Master Transfer  SPISelect=SPI_A  ClockPolarity=Rising_edge  ClockPhase=Delay_half_cycle  SPIModule=uint32(0)  Mode=Master  BusSpeed=uint32(1000000)  FirstBitToTransfer=Most significant bit (MSB)  ClockMode=0  BlockFunction=Transfer  EnableRegisterAddress=off  RegisterAddress=0  OutputDataType=int8  OutputDataLength=1  DataBits=8  UseCustomSSPin=Explicit GPIO calls  ActiveLowSSPin=Active low  Pin=124
      settings: SourceProductBaseCode=TIC2000
  Terminator : Terminator
  wires:
  cmd/1 -> SPI Master Transfer/1
  SPI Master Transfer/1 -> Terminator/1

== system c2837xD_lcd_display/Initialization/OscStart/Subsystem/SendData ==
  Data : Inport
  function : TriggerPort  TriggerType=function-call  VariantControl=Variant
  SPI Master Transfer : c280xlib/SPI Master Transfer  SPISelect=SPI_A  ClockPolarity=Rising_edge  ClockPhase=Delay_half_cycle  SPIModule=uint32(0)  Mode=Master  BusSpeed=uint32(1000000)  FirstBitToTransfer=Most significant bit (MSB)  ClockMode=0  BlockFunction=Transfer  EnableRegisterAddress=off  RegisterAddress=0  OutputDataType=int8  OutputDataLength=1  DataBits=8  UseCustomSSPin=Explicit GPIO calls  ActiveLowSSPin=Active low  Pin=124
      settings: SourceProductBaseCode=TIC2000
  Terminator : Terminator
  wires:
  Data/1 -> SPI Master Transfer/1
  SPI Master Transfer/1 -> Terminator/1

== system c2837xD_lcd_display/Initialization/OscStart/Subsystem/SetCmd ==
  function : TriggerPort  TriggerType=function-call  VariantControl=Variant
  Constant : Constant  Value=0  SampleTime=-1
  Digital Output : c2837xDlib/Digital Output  GPIO_Number=GPIO16~GPIO23  GPIO_Bit0=off  GPIO_BIT0_Toggle=off  GPIO_Bit1=off  GPIO_BIT1_Toggle=off  GPIO_Bit2=off  GPIO_BIT2_Toggle=off  GPIO_Bit3=off  GPIO_BIT3_Toggle=off  GPIO_Bit4=off  GPIO_BIT4_Toggle=off  GPIO_Bit5=off  GPIO_BIT5_Toggle=off  GPIO_Bit6=on  GPIO_BIT6_Toggle=off  GPIO_Bit7=off  GPIO_BIT7_Toggle=off
      settings: SourceProductBaseCode=TIC2000
  wires:
  Constant/1 -> Digital Output/1

== system c2837xD_lcd_display/Initialization/OscStart/Subsystem/SetData ==
  function : TriggerPort  TriggerType=function-call  VariantControl=Variant
  Constant1 : Constant  SampleTime=-1
  Digital Output1 : c2837xDlib/Digital Output  GPIO_Number=GPIO16~GPIO23  GPIO_Bit0=off  GPIO_BIT0_Toggle=off  GPIO_Bit1=off  GPIO_BIT1_Toggle=off  GPIO_Bit2=off  GPIO_BIT2_Toggle=off  GPIO_Bit3=off  GPIO_BIT3_Toggle=off  GPIO_Bit4=off  GPIO_BIT4_Toggle=off  GPIO_Bit5=off  GPIO_BIT5_Toggle=off  GPIO_Bit6=on  GPIO_BIT6_Toggle=off  GPIO_Bit7=off  GPIO_BIT7_Toggle=off
      settings: SourceProductBaseCode=TIC2000
  wires:
  Constant1/1 -> Digital Output1/1

== system c2837xD_lcd_display/Initialization/Reset/COMMAND/System Outputs ==

== system c2837xD_lcd_display/Initialization/Reset/DATA/System Outputs ==

== system c2837xD_lcd_display/Initialization/Reset/DeselectLCD/System Outputs1 ==

== system c2837xD_lcd_display/Initialization/Reset/LCD RESET/System Outputs ==

== system c2837xD_lcd_display/Initialization/Reset/SelectLCD/System Outputs1 ==

== system c2837xD_lcd_display/Initialization/SleepMode/Subsystem/SendCommand ==
  cmd : Inport
  function : TriggerPort  TriggerType=function-call  VariantControl=Variant
  SPI Master Transfer : c280xlib/SPI Master Transfer  SPISelect=SPI_A  ClockPolarity=Rising_edge  ClockPhase=Delay_half_cycle  SPIModule=uint32(0)  Mode=Master  BusSpeed=uint32(1000000)  FirstBitToTransfer=Most significant bit (MSB)  ClockMode=0  BlockFunction=Transfer  EnableRegisterAddress=off  RegisterAddress=0  OutputDataType=int8  OutputDataLength=1  DataBits=8  UseCustomSSPin=Explicit GPIO calls  ActiveLowSSPin=Active low  Pin=124
      settings: SourceProductBaseCode=TIC2000
  Terminator : Terminator
  wires:
  cmd/1 -> SPI Master Transfer/1
  SPI Master Transfer/1 -> Terminator/1

== system c2837xD_lcd_display/Initialization/SleepMode/Subsystem/SendData ==
  Data : Inport
  function : TriggerPort  TriggerType=function-call  VariantControl=Variant
  SPI Master Transfer : c280xlib/SPI Master Transfer  SPISelect=SPI_A  ClockPolarity=Rising_edge  ClockPhase=Delay_half_cycle  SPIModule=uint32(0)  Mode=Master  BusSpeed=uint32(1000000)  FirstBitToTransfer=Most significant bit (MSB)  ClockMode=0  BlockFunction=Transfer  EnableRegisterAddress=off  RegisterAddress=0  OutputDataType=int8  OutputDataLength=1  DataBits=8  UseCustomSSPin=Explicit GPIO calls  ActiveLowSSPin=Active low  Pin=124
      settings: SourceProductBaseCode=TIC2000
  Terminator : Terminator
  wires:
  Data/1 -> SPI Master Transfer/1
  SPI Master Transfer/1 -> Terminator/1

== system c2837xD_lcd_display/Initialization/SleepMode/Subsystem/SetCmd ==
  function : TriggerPort  TriggerType=function-call  VariantControl=Variant
  Constant : Constant  Value=0  SampleTime=-1
  Digital Output : c2837xDlib/Digital Output  GPIO_Number=GPIO16~GPIO23  GPIO_Bit0=off  GPIO_BIT0_Toggle=off  GPIO_Bit1=off  GPIO_BIT1_Toggle=off  GPIO_Bit2=off  GPIO_BIT2_Toggle=off  GPIO_Bit3=off  GPIO_BIT3_Toggle=off  GPIO_Bit4=off  GPIO_BIT4_Toggle=off  GPIO_Bit5=off  GPIO_BIT5_Toggle=off  GPIO_Bit6=on  GPIO_BIT6_Toggle=off  GPIO_Bit7=off  GPIO_BIT7_Toggle=off
      settings: SourceProductBaseCode=TIC2000
  wires:
  Constant/1 -> Digital Output/1

== system c2837xD_lcd_display/Initialization/SleepMode/Subsystem/SetData ==
  function : TriggerPort  TriggerType=function-call  VariantControl=Variant
  Constant1 : Constant  SampleTime=-1
  Digital Output1 : c2837xDlib/Digital Output  GPIO_Number=GPIO16~GPIO23  GPIO_Bit0=off  GPIO_BIT0_Toggle=off  GPIO_Bit1=off  GPIO_BIT1_Toggle=off  GPIO_Bit2=off  GPIO_BIT2_Toggle=off  GPIO_Bit3=off  GPIO_BIT3_Toggle=off  GPIO_Bit4=off  GPIO_BIT4_Toggle=off  GPIO_Bit5=off  GPIO_BIT5_Toggle=off  GPIO_Bit6=on  GPIO_BIT6_Toggle=off  GPIO_Bit7=off  GPIO_BIT7_Toggle=off
      settings: SourceProductBaseCode=TIC2000
  wires:
  Constant1/1 -> Digital Output1/1

== system c2837xD_lcd_display/Initialization/VCOM_OTP_1_REG/Subsystem/SendCommand ==
  cmd : Inport
  function : TriggerPort  TriggerType=function-call  VariantControl=Variant
  SPI Master Transfer : c280xlib/SPI Master Transfer  SPISelect=SPI_A  ClockPolarity=Rising_edge  ClockPhase=Delay_half_cycle  SPIModule=uint32(0)  Mode=Master  BusSpeed=uint32(1000000)  FirstBitToTransfer=Most significant bit (MSB)  ClockMode=0  BlockFunction=Transfer  EnableRegisterAddress=off  RegisterAddress=0  OutputDataType=int8  OutputDataLength=1  DataBits=8  UseCustomSSPin=Explicit GPIO calls  ActiveLowSSPin=Active low  Pin=124
      settings: SourceProductBaseCode=TIC2000
  Terminator : Terminator
  wires:
  cmd/1 -> SPI Master Transfer/1
  SPI Master Transfer/1 -> Terminator/1

== system c2837xD_lcd_display/Initialization/VCOM_OTP_1_REG/Subsystem/SendData ==
  Data : Inport
  function : TriggerPort  TriggerType=function-call  VariantControl=Variant
  SPI Master Transfer : c280xlib/SPI Master Transfer  SPISelect=SPI_A  ClockPolarity=Rising_edge  ClockPhase=Delay_half_cycle  SPIModule=uint32(0)  Mode=Master  BusSpeed=uint32(1000000)  FirstBitToTransfer=Most significant bit (MSB)  ClockMode=0  BlockFunction=Transfer  EnableRegisterAddress=off  RegisterAddress=0  OutputDataType=int8  OutputDataLength=1  DataBits=8  UseCustomSSPin=Explicit GPIO calls  ActiveLowSSPin=Active low  Pin=124
      settings: SourceProductBaseCode=TIC2000
  Terminator : Terminator
  wires:
  Data/1 -> SPI Master Transfer/1
  SPI Master Transfer/1 -> Terminator/1

== system c2837xD_lcd_display/Initialization/VCOM_OTP_1_REG/Subsystem/SetCmd ==
  function : TriggerPort  TriggerType=function-call  VariantControl=Variant
  Constant : Constant  Value=0  SampleTime=-1
  Digital Output : c2837xDlib/Digital Output  GPIO_Number=GPIO16~GPIO23  GPIO_Bit0=off  GPIO_BIT0_Toggle=off  GPIO_Bit1=off  GPIO_BIT1_Toggle=off  GPIO_Bit2=off  GPIO_BIT2_Toggle=off  GPIO_Bit3=off  GPIO_BIT3_Toggle=off  GPIO_Bit4=off  GPIO_BIT4_Toggle=off  GPIO_Bit5=off  GPIO_BIT5_Toggle=off  GPIO_Bit6=on  GPIO_BIT6_Toggle=off  GPIO_Bit7=off  GPIO_BIT7_Toggle=off
      settings: SourceProductBaseCode=TIC2000
  wires:
  Constant/1 -> Digital Output/1
